simulink model "red_y_planta_LINEALES"  (R2023b)
settings: Solver=ode45  StartTime=0.0  StopTime=5000  RelTol=1e-3
values from neighbouring files (symbols this model uses):
  D = 0    [control_pid_tuning.m]
  muT = 2.28832038256e-05    [LIN_prueba1.mat]    (also in LINnet_10_dataset14400.mat = 2.29669959879e-05; LINnet_20_dataset14400.mat = 2.28411149828e-05; entrenar_sistema_lineal_mas_no_lineal.m = mean(T); experimentos_identificacion.m = mean(T))
  muX = [0.00195137264409 0.00195123975627 0.00195110674472 0.00195097362517 0.00195084041422 0.00195070712945 0.00195057378941 0.00195044041376 0.00199709257249]    [LIN_prueba1.mat]    (also in LINnet_10_dataset14400.mat = [0.00195056060449 0.00195042737275 0.00199710863997]; LINnet_20_dataset14400.mat = [0.0019516426524 0.00195151000821 0.00195137721131 0.0019512; entrenar_sistema_lineal_mas_no_lineal.m = mean(X, 1); experimentos_identificacion.m = mean(X, 1))
  ny = 8    [LIN_prueba1.mat]    (also in LINnet_10_dataset14400.mat = 2; LINnet_20_dataset14400.mat = 10; entrenar_datasets.m = 10; entrenar_sistema_lineal_mas_no_lineal.m)
  sigT = 0.000100672763692    [LIN_prueba1.mat]    (also in LINnet_10_dataset14400.mat = 0.000100741004876; LINnet_20_dataset14400.mat = 0.000100616353545; entrenar_sistema_lineal_mas_no_lineal.m = 1; experimentos_identificacion.m = 1)
  sigX = [0.000218672390723 0.000219272765797 0.00021987238908 0.000220471128037 0.000221068843335 0.000221665388538 0.000222260609795 0.000222854345519 9.66176597141e-05]    [LIN_prueba1.mat]    (also in LINnet_10_dataset14400.mat = [0.000222215232754 0.000222808821935 9.66007318408e-05]; LINnet_20_dataset14400.mat = [0.000217484635478 0.000218086192323 0.000218687243085 0.000; entrenar_sistema_lineal_mas_no_lineal.m = std(X, 0, 1); experimentos_identificacion.m = std(X, 0, 1))
libraries: neural x10, simulink x2
settings Model: Creator=q  LastModifiedBy=q

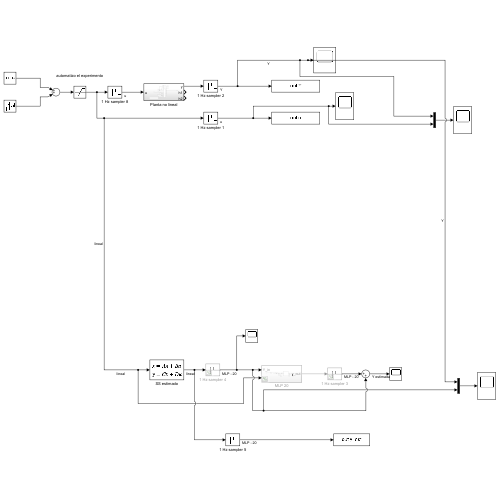
[thumbnail: Simulink's stored preview of the top-level diagram]
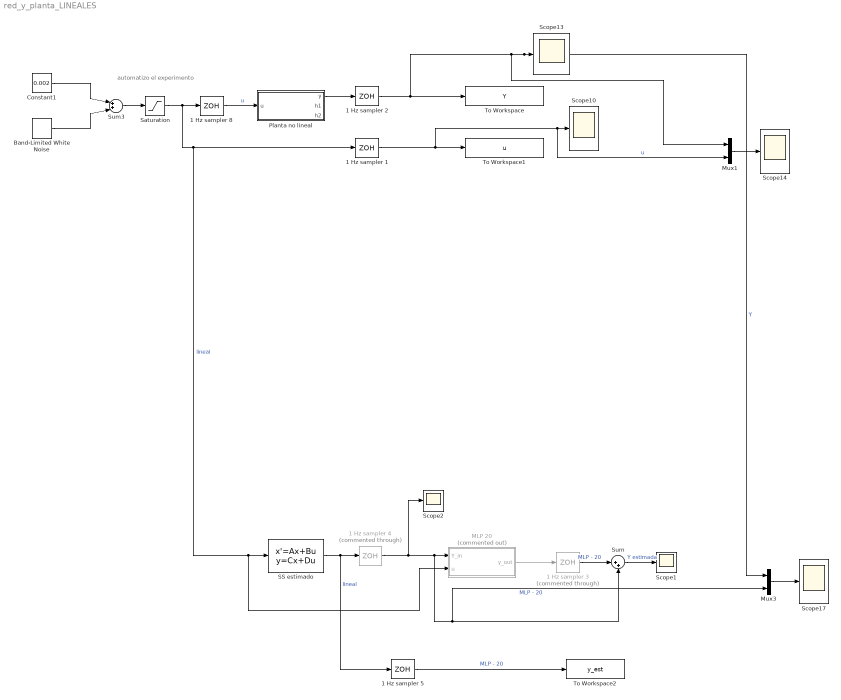
== system red_y_planta_LINEALES ==
  note: automatizo el experimento
  1 Hz sampler {1..2,5,8} (4 alike) : ZeroOrderHold
  1 Hz sampler 3 : ZeroOrderHold  Commented=through
  1 Hz sampler 4 : ZeroOrderHold  Commented=through
  Band-Limited White Noise : simulink/Sources/Band-Limited White Noise  Cov=[0.000002]  Ts=150  seed=[23341]
  Constant1 : Constant  Value=0.002
  MLP 20 : Subsystem  Commented=on
  Mux1 : Mux  Inputs=2
  Mux3 : Mux  Inputs=2
  Planta no lineal : Subsystem
  SS estimado : StateSpace  A=[-0.023375234759513,0.035713459182280;0.016442055191371,-0.031577082096728]  B=[2.537448139699421;-1.771387482474186]  C=[0.008723840649702,0.012539591066566]  D=0  InitialCondition=0
  Saturation : Saturate  UpperLimit=0.0022  LowerLimit=0.0018
  Scope{1..2,10,13..14,17} (6 alike) : Scope
  Sum : Sum  Inputs=|++
  Sum3 : Sum  Inputs=|++|
  To Workspace : ToWorkspace  VariableName=Y  SampleTime=1
  To Workspace1 : ToWorkspace  VariableName=u  SampleTime=1
  To Workspace2 : ToWorkspace  VariableName=y_est  SampleTime=-1
  wires:
  Planta no lineal/1(y) -> 1 Hz sampler 2/1
  Constant1/1 -> Sum3/1
  Sum3/1 -> Saturation/1
  Band-Limited White Noise/1 -> Sum3/2
  1 Hz sampler 2/1 -> Mux3/1, Scope13/1, Mux1/1, To Workspace/1  "Y"
  1 Hz sampler 1/1 -> Mux1/2, Scope10/1, To Workspace1/1  "u"
  MLP 20/1(y_out) -> 1 Hz sampler 3/1
  Mux1/1 -> Scope14/1
  1 Hz sampler 8/1 -> Planta no lineal/1(u)  "u"
  Mux3/1 -> Scope17/1
  Saturation/1 -> 1 Hz sampler 8/1, MLP 20/2(u), SS estimado/1, 1 Hz sampler 1/1  "lineal"
  SS estimado/1 -> 1 Hz sampler 5/1, 1 Hz sampler 4/1  "lineal"
  1 Hz sampler 4/1 -> Scope2/1, Mux3/2, Sum/2, MLP 20/1(Y_in)  "MLP - 20"
  1 Hz sampler 3/1 -> Sum/1  "MLP - 20"
  Sum/1 -> Scope1/1  "Y estimada"
  1 Hz sampler 5/1 -> To Workspace2/1  "MLP - 20"

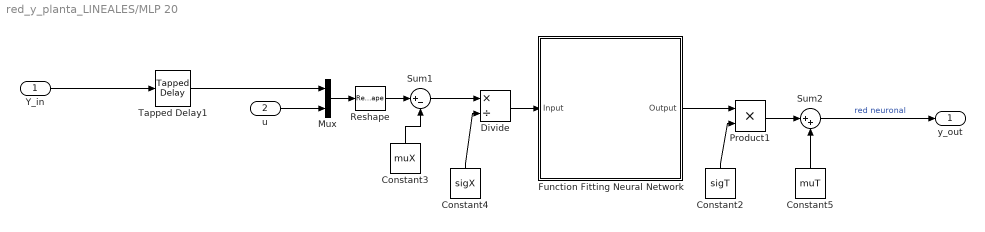
== system red_y_planta_LINEALES/MLP 20 ==
  Y_in : Inport
  u : Inport  Port=2
  Constant2 : Constant  Value=sigT
  Constant3 : Constant  Value=muX
  Constant4 : Constant  Value=sigX
  Constant5 : Constant  Value=muT
  Divide : Product  Inputs=*/
  Function Fitting Neural Network : Subsystem
      mask help: Function Fitting Neural Network
      mask Display: e = 0.06;c1 = [120 150 230]/255;c2 = ([120 150 230]+0)/383;c3 = ([120 150 230]+128)/383;patch([0 1 1 0],[0 0 1 1],c1);patch([0 1 1 1-e 1-e 0+e],[0 0 1 1-e 0+e 0+e],c2);patch([0 0 1 1-e 0+e 0+e],[0 1 1 1-e 1-e 0+e],c3);plot([0 1 1 0 0],[0 0 1 1 0]);fprintf('NNET');port_label('input',1,' Input');port_label('output',1,'Output ');
  Mux : Mux  Inputs=2
  Product1 : Product
  Reshape : Reshape  OutputDimensionality=Column vector (2-D)
  Sum1 : Sum  Inputs=|+-
  Sum2 : Sum  Inputs=|++
  Tapped Delay1 : simulink/Discrete/Tapped Delay  vinit=0  samptime=1  NumDelays=ny  DelayOrder=Newest  includeCurrent=off
  y_out : Outport
  wires:
  Constant3/1 -> Sum1/2
  Constant4/1 -> Divide/2
  Mux/1 -> Reshape/1
  Tapped Delay1/1 -> Mux/1
  Sum1/1 -> Divide/1
  Constant5/1 -> Sum2/2
  Reshape/1 -> Sum1/1
  Product1/1 -> Sum2/1
  Constant2/1 -> Product1/2
  Y_in/1 -> Tapped Delay1/1
  u/1 -> Mux/2
  Sum2/1 -> y_out/1  "red neuronal"
  Function Fitting Neural Network/1(Output) -> Product1/1
  Divide/1 -> Function Fitting Neural Network/1(Input)

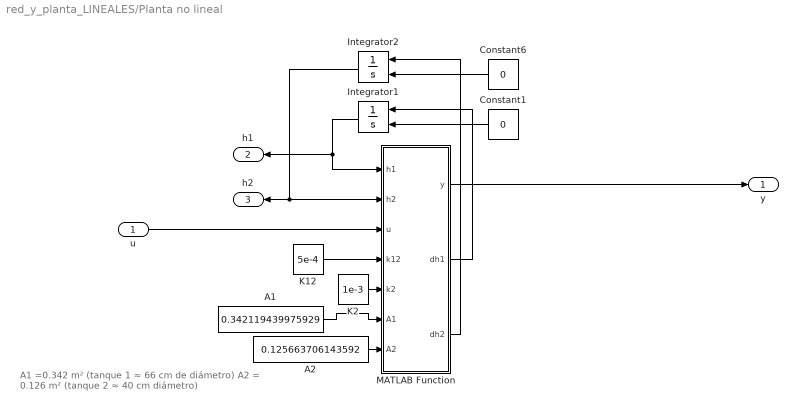
== system red_y_planta_LINEALES/Planta no lineal ==
  note: A1 =0.342   m²   (tanque 1 ≈ 66 cm de diámetro)
      | A2 = 0.126   m²   (tanque 2 ≈ 40 cm diámetro)
  u : Inport
  A1 : Constant  Value=0.342119439975929
  A2 : Constant  Value=0.125663706143592
  Constant1 : Constant  Value=0
  Constant6 : Constant  Value=0
  Integrator1 : Integrator  InitialConditionSource=external
  Integrator2 : Integrator  InitialConditionSource=external
  K12 : Constant  Value=5e-4
  K2 : Constant  Value=1e-3
  MATLAB Function : MATLAB Function  TreatAsAtomicUnit=on
  y : Outport
  h1 : Outport  Port=2
  h2 : Outport  Port=3
  wires:
  K2/1 -> MATLAB Function/5(k2)
  MATLAB Function/3(dh2) -> Integrator2/1
  MATLAB Function/2(dh1) -> Integrator1/1
  Integrator1/1 -> h1/1, MATLAB Function/1(h1)
  Constant6/1 -> Integrator2/2
  A2/1 -> MATLAB Function/7(A2)
  Constant1/1 -> Integrator1/2
  u/1 -> MATLAB Function/3(u)
  MATLAB Function/1(y) -> y/1
  Integrator2/1 -> h2/1, MATLAB Function/2(h2)
  A1/1 -> MATLAB Function/6(A1)
  K12/1 -> MATLAB Function/4(k12)

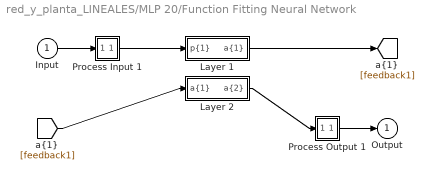
== system red_y_planta_LINEALES/MLP 20/Function Fitting Neural Network ==
  Input : Inport  PortDimensions=9
      mask Display: e = 0.06;c1 = [120 230 180]/255;c2 = ([120 230 180]+0)/(256+128);c3 = ([120 230 180]+128)/(256+128);patch([0 1 1 0],[0 0 1 1],c1);patch([0 1 1 1-e 1-e 0+e],[0 0 1 1-e 0+e 0+e],c2);patch([0 0 1 1-e 0+e 0+e],[0 1 1 1-e 1-e 0+e],c3);plot([0 1 1 0 0],[0 0 1 1 0]);
  Layer 1 : Subsystem
      mask Display: e = 0.06;c1 = [120 150 230]/255;c2 = ([120 150 230]+0)/383;c3 = ([120 150 230]+128)/383;patch([0 1 1 0],[0 0 1 1],c1);patch([0 1 1 1-e 1-e 0+e],[0 0 1 1-e 0+e 0+e],c2);patch([0 0 1 1-e 0+e 0+e],[0 1 1 1-e 1-e 0+e],c3);plot([0 1 1 0 0],[0 0 1 1 0]);
  Layer 2 : Subsystem
      mask Display: e = 0.06;c1 = [120 150 230]/255;c2 = ([120 150 230]+0)/383;c3 = ([120 150 230]+128)/383;patch([0 1 1 0],[0 0 1 1],c1);patch([0 1 1 1-e 1-e 0+e],[0 0 1 1-e 0+e 0+e],c2);patch([0 0 1 1-e 0+e 0+e],[0 1 1 1-e 1-e 0+e],c3);plot([0 1 1 0 0],[0 0 1 1 0]);
  Process Input 1 : Subsystem
      mask Display: e = 0.06;c1 = [120 150 230]/255;c2 = ([120 150 230]+0)/383;c3 = ([120 150 230]+128)/383;patch([0 1 1 0],[0 0 1 1],c1);patch([0 1 1 1-e 1-e 0+e],[0 0 1 1-e 0+e 0+e],c2);patch([0 0 1 1-e 0+e 0+e],[0 1 1 1-e 1-e 0+e],c3);plot([0 1 1 0 0],[0 0 1 1 0]);
  Process Output 1 : Subsystem
      mask Display: e = 0.06;c1 = [120 150 230]/255;c2 = ([120 150 230]+0)/383;c3 = ([120 150 230]+128)/383;patch([0 1 1 0],[0 0 1 1],c1);patch([0 1 1 1-e 1-e 0+e],[0 0 1 1-e 0+e 0+e],c2);patch([0 0 1 1-e 0+e 0+e],[0 1 1 1-e 1-e 0+e],c3);plot([0 1 1 0 0],[0 0 1 1 0]);
  Output : Outport  InitialOutput=0
      mask Display: e = 0.06;c1 = [120 230 180]/255;c2 = ([120 230 180]+0)/(256+128);c3 = ([120 230 180]+128)/(256+128);patch([0 1 1 0],[0 0 1 1],c1);patch([0 1 1 1-e 1-e 0+e],[0 0 1 1-e 0+e 0+e],c2);patch([0 0 1 1-e 0+e 0+e],[0 1 1 1-e 1-e 0+e],c3);plot([0 1 1 0 0],[0 0 1 1 0]);
  wires:
  Input/1 -> Process Input 1/1(x)
  Process Output 1/1(y) -> Output/1
  Process Input 1/1(p) -> Layer 1/1("p{1}")
  Layer 1/1("a{1}") -> [feedback1]
  [feedback1] -> Layer 2/1("a{1} ")
  Layer 2/1("a{2}") -> Process Output 1/1(a)

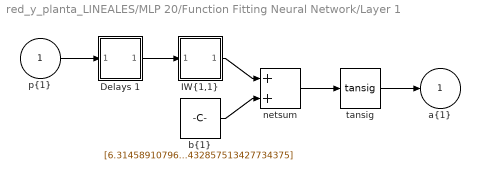
== system red_y_planta_LINEALES/MLP 20/Function Fitting Neural Network/Layer 1 ==
  "p{1}" : Inport  PortDimensions=9
      mask Display: e = 0.06;c1 = [120 230 180]/255;c2 = ([120 230 180]+0)/(256+128);c3 = ([120 230 180]+128)/(256+128);patch([0 1 1 0],[0 0 1 1],c1);patch([0 1 1 1-e 1-e 0+e],[0 0 1 1-e 0+e 0+e],c2);patch([0 0 1 1-e 0+e 0+e],[0 1 1 1-e 1-e 0+e],c3);plot([0 1 1 0 0],[0 0 1 1 0]);
  Delays 1 : Subsystem
      mask Display: e = 0.06;c1 = [120 150 230]/255;c2 = ([120 150 230]+0)/383;c3 = ([120 150 230]+128)/383;patch([0 1 1 0],[0 0 1 1],c1);patch([0 1 1 1-e 1-e 0+e],[0 0 1 1-e 0+e 0+e],c2);patch([0 0 1 1-e 0+e 0+e],[0 1 1 1-e 1-e 0+e],c3);plot([0 1 1 0 0],[0 0 1 1 0]);disp('0');
  "IW{1,1}" : Subsystem
      mask Display: e = 0.06;c1 = [120 150 230]/255;c2 = ([120 150 230]+0)/383;c3 = ([120 150 230]+128)/383;patch([0 1 1 0],[0 0 1 1],c1);patch([0 1 1 1-e 1-e 0+e],[0 0 1 1-e 0+e 0+e],c2);patch([0 0 1 1-e 0+e 0+e],[0 1 1 1-e 1-e 0+e],c3);plot([0 1 1 0 0],[0 0 1 1 0]);disp('W');
  "b{1}" : Constant  Value=[6.31458910796001493537232818198390305042266845703125;-5.93087564493986807434566799202002584934234619140625;-7.6334509314276264291265761130489408969879150390625;0.68662727385751531894442223347141407430171966552734375;-2.607626162609329778518940656795166432857513427734375]
      mask Display: e = 0.06;c1 = [120 150 230]/255;c2 = ([120 150 230]+0)/383;c3 = ([120 150 230]+128)/383;patch([0 1 1 0],[0 0 1 1],c1);patch([0 1 1 1-e 1-e 0+e],[0 0 1 1-e 0+e 0+e],c2);patch([0 0 1 1-e 0+e 0+e],[0 1 1 1-e 1-e 0+e],c3);plot([0 1 1 0 0],[0 0 1 1 0]);disp('b');
  netsum : Sum  Inputs=2  InputSameDT=on  SaturateOnIntegerOverflow=on  OutDataTypeStr=Inherit: Same as first input
      mask Display: e = 0.06;c1 = [120 150 230]/255;c2 = ([120 150 230]+0)/383;c3 = ([120 150 230]+128)/383;patch([0 1 1 0],[0 0 1 1],c1);patch([0 1 1 1-e 1-e 0+e],[0 0 1 1-e 0+e 0+e],c2);patch([0 0 1 1-e 0+e 0+e],[0 1 1 1-e 1-e 0+e],c3);plot([0 1 1 0 0],[0 0 1 1 0]);disp('+');
  tansig : neural/Transfer Functions/tansig
  "a{1}" : Outport  InitialOutput=[0;0;0;0;0]
      mask Display: e = 0.06;c1 = [120 230 180]/255;c2 = ([120 230 180]+0)/(256+128);c3 = ([120 230 180]+128)/(256+128);patch([0 1 1 0],[0 0 1 1],c1);patch([0 1 1 1-e 1-e 0+e],[0 0 1 1-e 0+e 0+e],c2);patch([0 0 1 1-e 0+e 0+e],[0 1 1 1-e 1-e 0+e],c3);plot([0 1 1 0 0],[0 0 1 1 0]);
  wires:
  "p{1}"/1 -> Delays 1/1("p{1}")
  Delays 1/1("pd{1,1}") -> "IW{1,1}"/1("pd{1,1}")
  "IW{1,1}"/1("iz{1,1}") -> netsum/1
  "b{1}"/1 -> netsum/2
  netsum/1 -> tansig/1
  tansig/1 -> "a{1}"/1

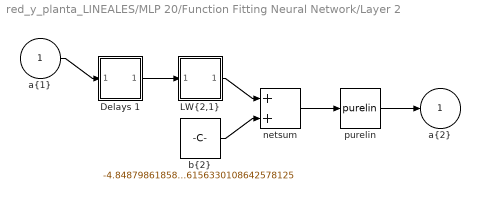
== system red_y_planta_LINEALES/MLP 20/Function Fitting Neural Network/Layer 2 ==
  "a{1} " : Inport  PortDimensions=5
      mask Display: e = 0.06;c1 = [120 230 180]/255;c2 = ([120 230 180]+0)/(256+128);c3 = ([120 230 180]+128)/(256+128);patch([0 1 1 0],[0 0 1 1],c1);patch([0 1 1 1-e 1-e 0+e],[0 0 1 1-e 0+e 0+e],c2);patch([0 0 1 1-e 0+e 0+e],[0 1 1 1-e 1-e 0+e],c3);plot([0 1 1 0 0],[0 0 1 1 0]);
  Delays 1 : Subsystem
      mask Display: e = 0.06;c1 = [120 150 230]/255;c2 = ([120 150 230]+0)/383;c3 = ([120 150 230]+128)/383;patch([0 1 1 0],[0 0 1 1],c1);patch([0 1 1 1-e 1-e 0+e],[0 0 1 1-e 0+e 0+e],c2);patch([0 0 1 1-e 0+e 0+e],[0 1 1 1-e 1-e 0+e],c3);plot([0 1 1 0 0],[0 0 1 1 0]);disp('0');
  "LW{2,1}" : Subsystem
      mask Display: e = 0.06;c1 = [120 150 230]/255;c2 = ([120 150 230]+0)/383;c3 = ([120 150 230]+128)/383;patch([0 1 1 0],[0 0 1 1],c1);patch([0 1 1 1-e 1-e 0+e],[0 0 1 1-e 0+e 0+e],c2);patch([0 0 1 1-e 0+e 0+e],[0 1 1 1-e 1-e 0+e],c3);plot([0 1 1 0 0],[0 0 1 1 0]);disp('W');
  "b{2}" : Constant  Value=-4.848798618586943831587632303126156330108642578125
      mask Display: e = 0.06;c1 = [120 150 230]/255;c2 = ([120 150 230]+0)/383;c3 = ([120 150 230]+128)/383;patch([0 1 1 0],[0 0 1 1],c1);patch([0 1 1 1-e 1-e 0+e],[0 0 1 1-e 0+e 0+e],c2);patch([0 0 1 1-e 0+e 0+e],[0 1 1 1-e 1-e 0+e],c3);plot([0 1 1 0 0],[0 0 1 1 0]);disp('b');
  netsum : Sum  Inputs=2  InputSameDT=on  SaturateOnIntegerOverflow=on  OutDataTypeStr=Inherit: Same as first input
      mask Display: e = 0.06;c1 = [120 150 230]/255;c2 = ([120 150 230]+0)/383;c3 = ([120 150 230]+128)/383;patch([0 1 1 0],[0 0 1 1],c1);patch([0 1 1 1-e 1-e 0+e],[0 0 1 1-e 0+e 0+e],c2);patch([0 0 1 1-e 0+e 0+e],[0 1 1 1-e 1-e 0+e],c3);plot([0 1 1 0 0],[0 0 1 1 0]);disp('+');
  purelin : neural/Transfer Functions/purelin
  "a{2}" : Outport  InitialOutput=0
      mask Display: e = 0.06;c1 = [120 230 180]/255;c2 = ([120 230 180]+0)/(256+128);c3 = ([120 230 180]+128)/(256+128);patch([0 1 1 0],[0 0 1 1],c1);patch([0 1 1 1-e 1-e 0+e],[0 0 1 1-e 0+e 0+e],c2);patch([0 0 1 1-e 0+e 0+e],[0 1 1 1-e 1-e 0+e],c3);plot([0 1 1 0 0],[0 0 1 1 0]);
  wires:
  "a{1} "/1 -> Delays 1/1("p{2}")
  Delays 1/1("pd{2,1}") -> "LW{2,1}"/1("ad{2,1}")
  "LW{2,1}"/1("lz{2,1}") -> netsum/1
  "b{2}"/1 -> netsum/2
  netsum/1 -> purelin/1
  purelin/1 -> "a{2}"/1

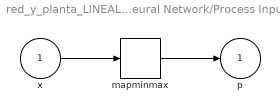
== system red_y_planta_LINEALES/MLP 20/Function Fitting Neural Network/Process Input 1 ==
  x : Inport  PortDimensions=9
      mask Display: e = 0.06;c1 = [120 230 180]/255;c2 = ([120 230 180]+0)/(256+128);c3 = ([120 230 180]+128)/(256+128);patch([0 1 1 0],[0 0 1 1],c1);patch([0 1 1 1-e 1-e 0+e],[0 0 1 1-e 0+e 0+e],c2);patch([0 0 1 1-e 0+e 0+e],[0 1 1 1-e 1-e 0+e],c3);plot([0 1 1 0 0],[0 0 1 1 0]);
  mapminmax : neural/Processing Functions/mapminmax  xmin=[-8.88927239990644402212183194933;-8.87246614958722723542905441718;-8.85480638077056703139078308595;-8.83624922575010529612882237416;-8.81674850487852346248018875485;-8.79625559966386560972750885412;-8.77471931840684860048895643558;-8.7520857538962832933293611859;-2.03992285746957069392237826833]  xmax=[0.750357120481400352574041789921;0.748908660218737032288061072904;0.747471228591012226694090259116;0.746045098133187756239692589588;0.744630554069939720740478605876;0.743227894810273292947044865286;0.741837432453449463487515913585;0.740459493305299587539991534868;2.10010704165808581578289704339]  ymin=-1  ymax=1
  p : Outport  PortDimensions=9
      mask Display: e = 0.06;c1 = [120 230 180]/255;c2 = ([120 230 180]+0)/(256+128);c3 = ([120 230 180]+128)/(256+128);patch([0 1 1 0],[0 0 1 1],c1);patch([0 1 1 1-e 1-e 0+e],[0 0 1 1-e 0+e 0+e],c2);patch([0 0 1 1-e 0+e 0+e],[0 1 1 1-e 1-e 0+e],c3);plot([0 1 1 0 0],[0 0 1 1 0]);
  wires:
  x/1 -> mapminmax/1
  mapminmax/1 -> p/1

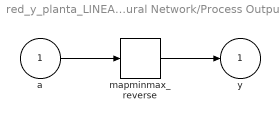
== system red_y_planta_LINEALES/MLP 20/Function Fitting Neural Network/Process Output 1 ==
  a : Inport  PortDimensions=1
      mask Display: e = 0.06;c1 = [120 230 180]/255;c2 = ([120 230 180]+0)/(256+128);c3 = ([120 230 180]+128)/(256+128);patch([0 1 1 0],[0 0 1 1],c1);patch([0 1 1 1-e 1-e 0+e],[0 0 1 1-e 0+e 0+e],c2);patch([0 0 1 1-e 0+e 0+e],[0 1 1 1-e 1-e 0+e],c3);plot([0 1 1 0 0],[0 0 1 1 0]);
  mapminmax_reverse : neural/Processing Functions/mapminmax_reverse  xmin=-0.286132263394823116442466925946  xmax=6.67855655179629703610544311232  ymin=-1  ymax=1
  y : Outport  PortDimensions=1
      mask Display: e = 0.06;c1 = [120 230 180]/255;c2 = ([120 230 180]+0)/(256+128);c3 = ([120 230 180]+128)/(256+128);patch([0 1 1 0],[0 0 1 1],c1);patch([0 1 1 1-e 1-e 0+e],[0 0 1 1-e 0+e 0+e],c2);patch([0 0 1 1-e 0+e 0+e],[0 1 1 1-e 1-e 0+e],c3);plot([0 1 1 0 0],[0 0 1 1 0]);
  wires:
  a/1 -> mapminmax_reverse/1
  mapminmax_reverse/1 -> y/1

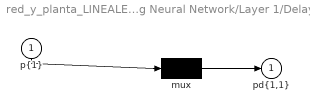
== system red_y_planta_LINEALES/MLP 20/Function Fitting Neural Network/Layer 1/Delays 1 ==
  "p{1}" : Inport  PortDimensions=9
      mask Display: e = 0.06;c1 = [120 230 180]/255;c2 = ([120 230 180]+0)/(256+128);c3 = ([120 230 180]+128)/(256+128);patch([0 1 1 0],[0 0 1 1],c1);patch([0 1 1 1-e 1-e 0+e],[0 0 1 1-e 0+e 0+e],c2);patch([0 0 1 1-e 0+e 0+e],[0 1 1 1-e 1-e 0+e],c3);plot([0 1 1 0 0],[0 0 1 1 0]);
  mux : Mux  Inputs=1
      mask Display: e = 0.06;c1 = [120 150 230]/255;c2 = ([120 150 230]+0)/383;c3 = ([120 150 230]+128)/383;patch([0 1 1 0],[0 0 1 1],c1);patch([0 1 1 1-e 1-e 0+e],[0 0 1 1-e 0+e 0+e],c2);patch([0 0 1 1-e 0+e 0+e],[0 1 1 1-e 1-e 0+e],c3);plot([0 1 1 0 0],[0 0 1 1 0]);disp('Mux')
  "pd{1,1}" : Outport
      mask Display: e = 0.06;c1 = [120 230 180]/255;c2 = ([120 230 180]+0)/(256+128);c3 = ([120 230 180]+128)/(256+128);patch([0 1 1 0],[0 0 1 1],c1);patch([0 1 1 1-e 1-e 0+e],[0 0 1 1-e 0+e 0+e],c2);patch([0 0 1 1-e 0+e 0+e],[0 1 1 1-e 1-e 0+e],c3);plot([0 1 1 0 0],[0 0 1 1 0]);
  wires:
  "p{1}"/1 -> mux/1
  mux/1 -> "pd{1,1}"/1

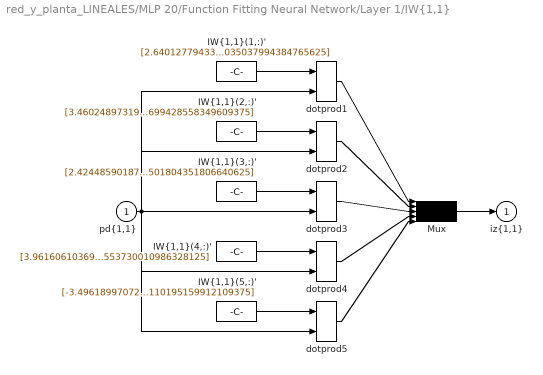
== system red_y_planta_LINEALES/MLP 20/Function Fitting Neural Network/Layer 1/IW{1,1} ==
  "pd{1,1}" : Inport  PortDimensions=9
      mask Display: e = 0.06;c1 = [120 230 180]/255;c2 = ([120 230 180]+0)/(256+128);c3 = ([120 230 180]+128)/(256+128);patch([0 1 1 0],[0 0 1 1],c1);patch([0 1 1 1-e 1-e 0+e],[0 0 1 1-e 0+e 0+e],c2);patch([0 0 1 1-e 0+e 0+e],[0 1 1 1-e 1-e 0+e],c3);plot([0 1 1 0 0],[0 0 1 1 0]);
  "IW{1,1}(1,:)'" : Constant  Value=[2.640127794338785971461902590817771852016448974609375;2.503301326205234378363684299984015524387359619140625;1.185597054578195308494059645454399287700653076171875;-0.1833928357562403521630045588608481921255588531494140625;-2.66067268070346418795679710456170141696929931640625;-2.11344875290565692438349287840537726879119873046875;-3.983663064070062542754158130264841020107269287109375;-4.27016799146210690452107883174903690814971923828125;-0.039972967475123723224417204846758977510035037994384765625]
      mask Display: e = 0.06;c1 = [120 150 230]/255;c2 = ([120 150 230]+0)/383;c3 = ([120 150 230]+128)/383;patch([0 1 1 0],[0 0 1 1],c1);patch([0 1 1 1-e 1-e 0+e],[0 0 1 1-e 0+e 0+e],c2);patch([0 0 1 1-e 0+e 0+e],[0 1 1 1-e 1-e 0+e],c3);plot([0 1 1 0 0],[0 0 1 1 0]);disp('Weights');
  "IW{1,1}(2,:)'" : Constant  Value=[3.46024897319468749401494278572499752044677734375;1.635426856731177824855194558040238916873931884765625;1.2587527315167268415763146549579687416553497314453125;0.174069269690645567205677934907726012170314788818359375;0.054678388832786813111841439649651874788105487823486328125;-0.421401729636686483981833362122415564954280853271484375;-0.003435089851788512664565455878573629888705909252166748046875;0.305883919086279709720344044399098493158817291259765625;0.0445332745022833653703031586701399646699428558349609375]
      mask Display: e = 0.06;c1 = [120 150 230]/255;c2 = ([120 150 230]+0)/383;c3 = ([120 150 230]+128)/383;patch([0 1 1 0],[0 0 1 1],c1);patch([0 1 1 1-e 1-e 0+e],[0 0 1 1-e 0+e 0+e],c2);patch([0 0 1 1-e 0+e 0+e],[0 1 1 1-e 1-e 0+e],c3);plot([0 1 1 0 0],[0 0 1 1 0]);disp('Weights');
  "IW{1,1}(3,:)'" : Constant  Value=[2.424485901874886994988855803967453539371490478515625;1.691943549894096232577567207044921815395355224609375;2.02451886142295567339033368625678122043609619140625;1.704194301862425486859820011886768043041229248046875;1.552239466010839397114295934443362057209014892578125;1.5120154980569135982904072079691104590892791748046875;2.754296519443241830771285094670020043849945068359375;2.755136878351687190757957068854011595249176025390625;-5.7719669151955432795375600107945501804351806640625]
      mask Display: e = 0.06;c1 = [120 150 230]/255;c2 = ([120 150 230]+0)/383;c3 = ([120 150 230]+128)/383;patch([0 1 1 0],[0 0 1 1],c1);patch([0 1 1 1-e 1-e 0+e],[0 0 1 1-e 0+e 0+e],c2);patch([0 0 1 1-e 0+e 0+e],[0 1 1 1-e 1-e 0+e],c3);plot([0 1 1 0 0],[0 0 1 1 0]);disp('Weights');
  "IW{1,1}(4,:)'" : Constant  Value=[3.961606103693756875117060189950279891490936279296875;4.28919505891390162588550083455629646778106689453125;3.129784687048297708855670862249098718166351318359375;0.91860267555272046013925546503742225468158721923828125;-0.274643878355773585209220755132264457643032073974609375;-1.8394808357765992656851494757574982941150665283203125;-3.925543230357173118960645297192968428134918212890625;-6.44221189089735890576093879644758999347686767578125;0.0037218433030262905447660415347854723222553730010986328125]
      mask Display: e = 0.06;c1 = [120 150 230]/255;c2 = ([120 150 230]+0)/383;c3 = ([120 150 230]+128)/383;patch([0 1 1 0],[0 0 1 1],c1);patch([0 1 1 1-e 1-e 0+e],[0 0 1 1-e 0+e 0+e],c2);patch([0 0 1 1-e 0+e 0+e],[0 1 1 1-e 1-e 0+e],c3);plot([0 1 1 0 0],[0 0 1 1 0]);disp('Weights');
  "IW{1,1}(5,:)'" : Constant  Value=[-3.496189970722433759675595865701325237751007080078125;-2.494917679692231882171427059802226722240447998046875;-1.4297320906464052736595249371021054685115814208984375;-0.002785129983921354017428750893259348231367766857147216796875;0.09281451281087453597518077685890602879226207733154296875;0.64473643297483296255023788035032339394092559814453125;0.9661608989678491798969162118737585842609405517578125;2.035258920400431659203377421363256871700286865234375;-3.46184700384318144728013066924177110195159912109375]
      mask Display: e = 0.06;c1 = [120 150 230]/255;c2 = ([120 150 230]+0)/383;c3 = ([120 150 230]+128)/383;patch([0 1 1 0],[0 0 1 1],c1);patch([0 1 1 1-e 1-e 0+e],[0 0 1 1-e 0+e 0+e],c2);patch([0 0 1 1-e 0+e 0+e],[0 1 1 1-e 1-e 0+e],c3);plot([0 1 1 0 0],[0 0 1 1 0]);disp('Weights');
  Mux : Mux  Inputs=5
      mask Display: e = 0.06;c1 = [120 150 230]/255;c2 = ([120 150 230]+0)/383;c3 = ([120 150 230]+128)/383;patch([0 1 1 0],[0 0 1 1],c1);patch([0 1 1 1-e 1-e 0+e],[0 0 1 1-e 0+e 0+e],c2);patch([0 0 1 1-e 0+e 0+e],[0 1 1 1-e 1-e 0+e],c3);plot([0 1 1 0 0],[0 0 1 1 0]);disp('Mux');
  dotprod{1..5} (5 alike) : neural/Weight Functions/dotprod
  "iz{1,1}" : Outport
      mask Display: e = 0.06;c1 = [120 230 180]/255;c2 = ([120 230 180]+0)/(256+128);c3 = ([120 230 180]+128)/(256+128);patch([0 1 1 0],[0 0 1 1],c1);patch([0 1 1 1-e 1-e 0+e],[0 0 1 1-e 0+e 0+e],c2);patch([0 0 1 1-e 0+e 0+e],[0 1 1 1-e 1-e 0+e],c3);plot([0 1 1 0 0],[0 0 1 1 0]);
  wires:
  "IW{1,1}(1,:)'"/1 -> dotprod1/1
  "pd{1,1}"/1 -> dotprod1/2, dotprod2/2, dotprod3/2, dotprod4/2, dotprod5/2
  dotprod1/1 -> Mux/1
  "IW{1,1}(2,:)'"/1 -> dotprod2/1
  dotprod2/1 -> Mux/2
  "IW{1,1}(3,:)'"/1 -> dotprod3/1
  dotprod3/1 -> Mux/3
  "IW{1,1}(4,:)'"/1 -> dotprod4/1
  dotprod4/1 -> Mux/4
  "IW{1,1}(5,:)'"/1 -> dotprod5/1
  dotprod5/1 -> Mux/5
  Mux/1 -> "iz{1,1}"/1

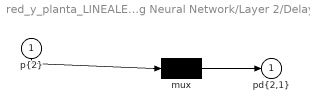
== system red_y_planta_LINEALES/MLP 20/Function Fitting Neural Network/Layer 2/Delays 1 ==
  "p{2}" : Inport  PortDimensions=5
      mask Display: e = 0.06;c1 = [120 230 180]/255;c2 = ([120 230 180]+0)/(256+128);c3 = ([120 230 180]+128)/(256+128);patch([0 1 1 0],[0 0 1 1],c1);patch([0 1 1 1-e 1-e 0+e],[0 0 1 1-e 0+e 0+e],c2);patch([0 0 1 1-e 0+e 0+e],[0 1 1 1-e 1-e 0+e],c3);plot([0 1 1 0 0],[0 0 1 1 0]);
  mux : Mux  Inputs=1
      mask Display: e = 0.06;c1 = [120 150 230]/255;c2 = ([120 150 230]+0)/383;c3 = ([120 150 230]+128)/383;patch([0 1 1 0],[0 0 1 1],c1);patch([0 1 1 1-e 1-e 0+e],[0 0 1 1-e 0+e 0+e],c2);patch([0 0 1 1-e 0+e 0+e],[0 1 1 1-e 1-e 0+e],c3);plot([0 1 1 0 0],[0 0 1 1 0]);disp('Mux')
  "pd{2,1}" : Outport
      mask Display: e = 0.06;c1 = [120 230 180]/255;c2 = ([120 230 180]+0)/(256+128);c3 = ([120 230 180]+128)/(256+128);patch([0 1 1 0],[0 0 1 1],c1);patch([0 1 1 1-e 1-e 0+e],[0 0 1 1-e 0+e 0+e],c2);patch([0 0 1 1-e 0+e 0+e],[0 1 1 1-e 1-e 0+e],c3);plot([0 1 1 0 0],[0 0 1 1 0]);
  wires:
  "p{2}"/1 -> mux/1
  mux/1 -> "pd{2,1}"/1

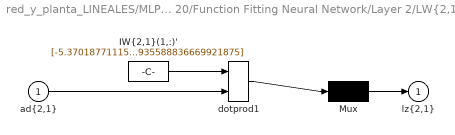
== system red_y_planta_LINEALES/MLP 20/Function Fitting Neural Network/Layer 2/LW{2,1} ==
  "ad{2,1}" : Inport  PortDimensions=5
      mask Display: e = 0.06;c1 = [120 230 180]/255;c2 = ([120 230 180]+0)/(256+128);c3 = ([120 230 180]+128)/(256+128);patch([0 1 1 0],[0 0 1 1],c1);patch([0 1 1 1-e 1-e 0+e],[0 0 1 1-e 0+e 0+e],c2);patch([0 0 1 1-e 0+e 0+e],[0 1 1 1-e 1-e 0+e],c3);plot([0 1 1 0 0],[0 0 1 1 0]);
  "IW{2,1}(1,:)'" : Constant  Value=[-5.37018771115907345148343665641732513904571533203125;-5.54184902528817691091944652725942432880401611328125;0.0861139173115501865840570872023818083107471466064453125;6.970614903620667490713458391837775707244873046875;-0.452969185730065226902496533512021414935588836669921875]
      mask Display: e = 0.06;c1 = [120 150 230]/255;c2 = ([120 150 230]+0)/383;c3 = ([120 150 230]+128)/383;patch([0 1 1 0],[0 0 1 1],c1);patch([0 1 1 1-e 1-e 0+e],[0 0 1 1-e 0+e 0+e],c2);patch([0 0 1 1-e 0+e 0+e],[0 1 1 1-e 1-e 0+e],c3);plot([0 1 1 0 0],[0 0 1 1 0]);disp('weights');
  Mux : Mux  Inputs=1
      mask Display: e = 0.06;c1 = [120 150 230]/255;c2 = ([120 150 230]+0)/383;c3 = ([120 150 230]+128)/383;patch([0 1 1 0],[0 0 1 1],c1);patch([0 1 1 1-e 1-e 0+e],[0 0 1 1-e 0+e 0+e],c2);patch([0 0 1 1-e 0+e 0+e],[0 1 1 1-e 1-e 0+e],c3);plot([0 1 1 0 0],[0 0 1 1 0]);disp('Mux');
  dotprod1 : neural/Weight Functions/dotprod
  "lz{2,1}" : Outport
      mask Display: e = 0.06;c1 = [120 230 180]/255;c2 = ([120 230 180]+0)/(256+128);c3 = ([120 230 180]+128)/(256+128);patch([0 1 1 0],[0 0 1 1],c1);patch([0 1 1 1-e 1-e 0+e],[0 0 1 1-e 0+e 0+e],c2);patch([0 0 1 1-e 0+e 0+e],[0 1 1 1-e 1-e 0+e],c3);plot([0 1 1 0 0],[0 0 1 1 0]);
  wires:
  "IW{2,1}(1,:)'"/1 -> dotprod1/1
  "ad{2,1}"/1 -> dotprod1/2
  dotprod1/1 -> Mux/1
  Mux/1 -> "lz{2,1}"/1

== matlab function red_y_planta_LINEALES/Planta no lineal/MATLAB Function ==
  data: h1 input; h2 input; y output; dh1 output; u input; k12 input; k2 input; A1 input; A2 input; dh2 output
function [y, dh1, dh2] = fcn(h1, h2, u, k12, k2, A1, A2)
g = 9.81;

delta_h = max(h1 - h2, 0);

q12 = k12 * sqrt(2 * g * delta_h); % caudal intermedio
q2  = k2  * sqrt(2 * g * max(h2, 0)); % caudal de salida

dh1 = (u - q12) / A1;
dh2 = (q12 - q2) / A2;

y = q2;

%el modelo asume flujo solo en un sentido

%se ignora inversión de flujo

%el sistema es válido para niveles positivos
